simulink model "sl_GTC_RRR"  (R2015b)
settings: Solver=ode45  StartTime=0.0  StopTime=2  MaxStep=1e-3  RelTol=1e-8
settings Model: ExtModeTrigMode=oneshot  ExtModeArmWhenConnect=off  Creator=Manuel G. Ortega  LastModifiedBy=Marco Montes Grova
settings DataIOCC: LimitDataPoints=off  SaveFormat=Array  SignalLoggingSaveFormat=ModelDataLogs
settings OptimizationCC: BooleanDataType=off  ExpressionDepthLimit=2147483647  InitFltsAndDblsToZero=on
settings DebuggingCC: SaveWithParameterizedLinksMsg=none  UnderspecifiedInitializationDetection=Classic  MergeDetectMultiDrivingBlocksExec=none  SignalResolutionControl=TryResolveAllWithWarning  MultiTaskDSMMsg=warning  MultiTaskCondExecSysMsg=none  FcnCallInpInsideContextMsg=EnableAllAsWarning  AllowSymbolicDim=on  StateNameClashWarn=warning
settings HardwareCC: ProdBitPerPointer=32  ProdLargestAtomicFloat=None  ProdIntDivRoundTo=Undefined  ProdEndianess=Unspecified  ProdWordSize=32  ProdHWDeviceType=32-bit Generic  TargetUnknown=on
settings GRTTargetCC: TargetFcnLib=ansi_tfl_tmw.mat  GeneratePreprocessorConditionals=Disable all  CombineOutputUpdateFcns=off  GRTInterface=on
settings ConfigComp: CovModelRefEnable=Off  CovSFcnEnable=off

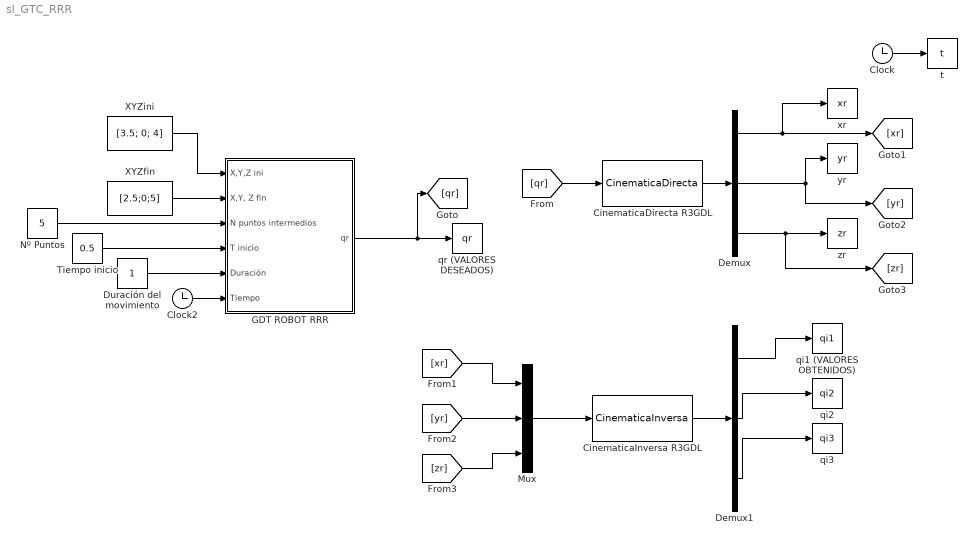
== system sl_GTC_RRR ==
  CinematicaDirecta R3GDL : MATLABFcn  MATLABFcn=CinematicaDirecta  OutputDimensions=3
  CinematicaInversa R3GDL : MATLABFcn  MATLABFcn=CinematicaInversa  OutputDimensions=3
  Clock : Clock
  Clock2 : Clock
  Demux : Demux  Outputs=3
  Demux1 : Demux  Outputs=3
  Duración del movimiento : Constant
  GDT ROBOT RRR : Subsystem
  Mux : Mux  Inputs=3
  Nº Puntos : Constant  Value=5
  Tiempo inicio : Constant  Value=0.5
  XYZfin : Constant  Value=[2.5;0;5]
  XYZini : Constant  Value=[3.5; 0; 4]
  qi1 (VALORES OBTENIDOS) : ToWorkspace  VariableName=qi1  SampleTime=-1
  "qi2 " : ToWorkspace  VariableName=qi2  SampleTime=-1
  "qi3 " : ToWorkspace  VariableName=qi3  SampleTime=-1
  qr (VALORES DESEADOS) : ToWorkspace  VariableName=qr  SampleTime=-1
  t : ToWorkspace  VariableName=t  SampleTime=-1
  xr : ToWorkspace  VariableName=xr  SampleTime=-1
  yr : ToWorkspace  VariableName=yr  SampleTime=-1
  zr : ToWorkspace  VariableName=zr  SampleTime=-1
  wires:
  Clock/1 -> t/1
  Clock2/1 -> GDT ROBOT RRR/6(Tiempo)
  Duración del movimiento/1 -> GDT ROBOT RRR/5(Duración)
  Tiempo inicio/1 -> GDT ROBOT RRR/4(T inicio)
  Nº Puntos/1 -> GDT ROBOT RRR/3(N puntos intermedios)
  XYZfin/1 -> GDT ROBOT RRR/2("X,Y, Z fin")
  XYZini/1 -> GDT ROBOT RRR/1(X,Y,Z ini)
  GDT ROBOT RRR/1(qr) -> qr (VALORES DESEADOS)/1, [qr]
  [qr] -> CinematicaDirecta R3GDL/1
  CinematicaDirecta R3GDL/1 -> Demux/1
  Demux/1 -> xr/1, [xr]
  Demux/2 -> [yr], yr/1
  Demux/3 -> [zr], zr/1
  [yr] -> Mux/2
  [zr] -> Mux/3
  [xr] -> Mux/1
  Mux/1 -> CinematicaInversa R3GDL/1
  CinematicaInversa R3GDL/1 -> Demux1/1
  Demux1/1 -> qi1 (VALORES OBTENIDOS)/1
  Demux1/3 -> "qi3 "/1
  Demux1/2 -> "qi2 "/1

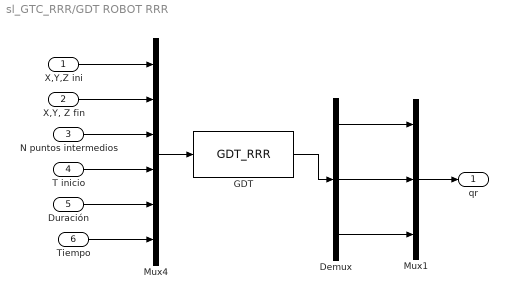
== system sl_GTC_RRR/GDT ROBOT RRR ==
  X,Y,Z ini : Inport
  "X,Y, Z fin" : Inport  Port=2
  N puntos intermedios : Inport  Port=3
  T inicio : Inport  Port=4
  Duración : Inport  Port=5
  Tiempo : Inport  Port=6
  Demux : Demux  Outputs=3
  "GDT " : MATLABFcn  MATLABFcn=GDT_RRR  OutputDimensions=3
  Mux1 : Mux  Inputs=3
  Mux4 : Mux  Inputs=6
  qr : Outport
  wires:
  Mux4/1 -> "GDT "/1
  X,Y,Z ini/1 -> Mux4/1
  "X,Y, Z fin"/1 -> Mux4/2
  N puntos intermedios/1 -> Mux4/3
  T inicio/1 -> Mux4/4
  Duración/1 -> Mux4/5
  Tiempo/1 -> Mux4/6
  "GDT "/1 -> Demux/1
  Demux/2 -> Mux1/2
  Demux/1 -> Mux1/1
  Demux/3 -> Mux1/3
  Mux1/1 -> qr/1
